simulink library "mech_stewart_controllers"  (Simulink 6.0)
settings: Solver=ode45  SolverMode=SingleTasking  StartTime=0.0  StopTime=10.0  RelTol=1e-3
undefined symbols (not defined in the file or in its folder): Ak, Aw, Bk, Bw, Ck, Cw, D, Dk, Dw, Kd, Ki, Kp, lower_leg_mass, nomForces, top_mass, upper_leg_mass
libraries: mech_stewart_controllers x1
settings Model: Creator=jwendlan  LastModifiedBy=batserve  ExtModeAutoUpdateStatusClock=off
settings OptimizationCC: BooleanDataType=off
settings DebuggingCC: SolverPrmCheckMsg=none
settings HardwareCC: TargetUnknown=on

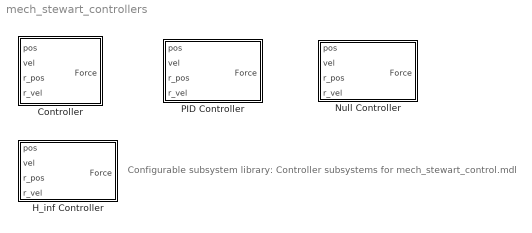
== system mech_stewart_controllers ==
  note: Configurable subsystem library:
      | Controller subsystems for
      | mech_stewart_control.mdl
  "Controller " : Subsystem  BlockChoice=Null Controller
      settings: TemplateBlock=self  MemberBlocks=H_inf Controller,Null Controller,PID Controller
  H_inf Controller : Subsystem
  Null Controller : Subsystem
  PID Controller : Subsystem

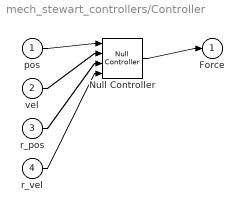
== system mech_stewart_controllers/Controller  ==
  pos : Inport  Port=1  LatchInput=off
  vel : Inport  Port=2  LatchInput=off
  r_pos : Inport  Port=3  LatchInput=off
  r_vel : Inport  Port=4  LatchInput=off
  Null Controller : mech_stewart_controllers/Null Controller
  Force : Outport
  wires:
  pos/1 -> Null Controller/1
  vel/1 -> Null Controller/2
  r_pos/1 -> Null Controller/3
  r_vel/1 -> Null Controller/4
  Null Controller/1 -> Force/1

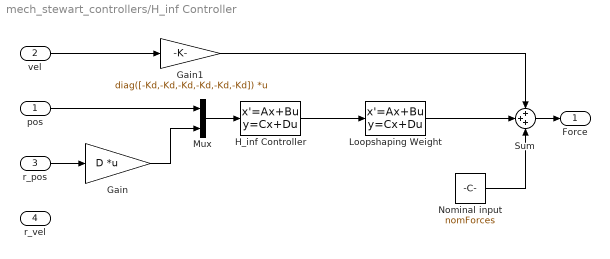
== system mech_stewart_controllers/H_inf Controller ==
  pos : Inport  Port=1  LatchInput=off
  vel : Inport  Port=2  LatchInput=off
  r_pos : Inport  Port=3  LatchInput=off
  r_vel : Inport  Port=4  LatchInput=off
  Gain : Gain  Gain=D  Multiplication=Matrix(K*u)  SaturateOnIntegerOverflow=on
  Gain1 : Gain  Gain=diag([-Kd,-Kd,-Kd,-Kd,-Kd,-Kd])  Multiplication=Matrix(K*u)  SaturateOnIntegerOverflow=on
  H_inf Controller : StateSpace  A=Ak  B=Bk  C=Ck  D=Dk
  Loopshaping Weight : StateSpace  A=Aw  B=Bw  C=Cw  D=Dw
  Mux : Mux  Inputs=2
  Nominal input : Constant  Value=nomForces
  Sum : Sum  Inputs=+++  SaturateOnIntegerOverflow=on  InputSameDT=on
  Force : Outport
  wires:
  Gain1/1 -> Sum/1
  Loopshaping Weight/1 -> Sum/2
  Nominal input/1 -> Sum/3
  vel/1 -> Gain1/1
  Gain/1 -> Mux/2
  r_pos/1 -> Gain/1
  Sum/1 -> Force/1
  pos/1 -> Mux/1
  Mux/1 -> H_inf Controller/1
  H_inf Controller/1 -> Loopshaping Weight/1

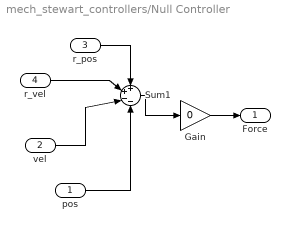
== system mech_stewart_controllers/Null Controller ==
  pos : Inport  Port=1  LatchInput=off
  vel : Inport  Port=2  LatchInput=off
  r_pos : Inport  Port=3  LatchInput=off
  r_vel : Inport  Port=4  LatchInput=off
  Gain : Gain  Gain=0
  Sum1 : Sum  Inputs=++--  SaturateOnIntegerOverflow=on  InputSameDT=on
  Force : Outport
  wires:
  Gain/1 -> Force/1
  Sum1/1 -> Gain/1
  pos/1 -> Sum1/4
  vel/1 -> Sum1/3
  r_pos/1 -> Sum1/1
  r_vel/1 -> Sum1/2

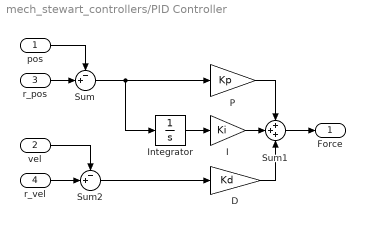
== system mech_stewart_controllers/PID Controller ==
  pos : Inport  Port=1  LatchInput=off
  vel : Inport  Port=2  LatchInput=off
  r_pos : Inport  Port=3  LatchInput=off
  r_vel : Inport  Port=4  LatchInput=off
  "   I" : Gain  Gain=Ki  SaturateOnIntegerOverflow=on
  D : Gain  Gain=Kd  SaturateOnIntegerOverflow=on
  Integrator : Integrator  InitialCondition=(upper_leg_mass+lower_leg_mass+(top_mass*1.3/6))*9.81/Ki  ZeroCross=off
  P : Gain  Gain=Kp  SaturateOnIntegerOverflow=on
  Sum : Sum  Inputs=-+|  SaturateOnIntegerOverflow=on  InputSameDT=on
  Sum1 : Sum  Inputs=+++  SaturateOnIntegerOverflow=on  InputSameDT=on
  Sum2 : Sum  Inputs=-+|  SaturateOnIntegerOverflow=on  InputSameDT=on
  Force : Outport
  wires:
  r_pos/1 -> Sum/2
  Sum1/1 -> Force/1
  pos/1 -> Sum/1
  D/1 -> Sum1/3
  Integrator/1 -> "   I"/1
  P/1 -> Sum1/1
  "   I"/1 -> Sum1/2
  Sum/1 -> Integrator/1, P/1
  vel/1 -> Sum2/1
  r_vel/1 -> Sum2/2
  Sum2/1 -> D/1
